simulink model "Planar_PIDC"  (R2022b)
settings: Solver=VariableStepAuto  StartTime=0.0  StopTime=40  RelTol=1e-3
values from neighbouring files (symbols this model uses):
  I = [1; 1; 1; 0.5; 0.5]*0.2    [RobDyn4link.m]
  l = [1; 1; 1; 1; 2]*0.2    [RobDyn4link.m]
  lc = l./2    [RobDyn4link.m]
  m = [1; 1; 1; 0.3; 0.3]*1    [RobDyn4link.m]
  q0 = [pi/2; -pi/4; -1*pi/6;-pi/12;0;]    [RobDyn4link.m]
  theta_max = [0.915*pi; 0.915*pi; 0.915*pi; 0.915*pi; 0.915*pi;]    [RobDyn4link.m]
  theta_min = [-0.915*pi; -0.915*pi; -0.915*pi; -0.915*pi; -0.915*pi;]    [RobDyn4link.m]
undefined symbols (not defined in the file or in its folder): DiscIntNeverNeededParam
(part 3 of 3)

== matlab function Planar_PIDC/Subsystem6/Subsystem/MATLAB Function ==
  data: theta input; M output; l input; lc input; I input; m input; Minv output
function [M,Minv] = fcn(theta,l,lc,I,m)
theta1 = theta(1); theta2 = theta(2); theta3 = theta(3); theta4 = theta(4); theta5 = theta(5);
% dtheta1 = dtheta(1); dtheta2 = dtheta(2); dtheta3 = dtheta(3); dtheta4 = dtheta(4); dtheta5 = dtheta(5);
I1 = I(1); I2 = I(2); I3 = I(3); I4 = I(4); I5 = I(5);
m1 = m(1); m2 = m(2); m3 = m(3); m4 = m(4); m5 = m(5);
l1 = l(1); l2 = l(2); l3 = l(3); l4 = l(4); l5 = l(5);
lc1 = lc(1); lc2 = lc(2); lc3 = lc(3); lc4 = lc(4); lc5 = lc(5);
% M = zeros(5,5);
% M(1,1) = I1 + I2 + I3 + I4 + I5 + l1^2*m2 + l1^2*m3 + l1^2*m4 + l2^2*m3 + l1^2*m5 + l2^2*m4 + l2^2*m5 + l3^2*m4 + l3^2*m5 + l4^2*m5 + lc1^2*m1 + lc2^2*m2 + lc3^2*m3 + lc4^2*m4 + lc5^2*m5 + 2*l1*lc5*m5*cos(theta2 + theta3 + theta4 + theta5) + 2*l1*l3*m4*cos(theta2 + theta3) + 2*l1*l3*m5*cos(theta2 + theta3) + 2*l2*l4*m5*cos(theta3 + theta4) + 2*l1*lc3*m3*cos(theta2 + theta3) + 2*l2*lc4*m4*cos(theta3 + theta4) + 2*l3*lc5*m5*cos(theta4 + theta5) + 2*l1*l2*m3*cos(theta2) + 2*l1*l2*m4*cos(theta2) + 2*l1*l2*m5*cos(theta2) + 2*l2*l3*m4*cos(theta3) + 2*l2*l3*m5*cos(theta3) + 2*l3*l4*m5*cos(theta4) + 2*l1*lc2*m2*cos(theta2) + 2*l2*lc3*m3*cos(theta3) + 2*l3*lc4*m4*cos(theta4) + 2*l4*lc5*m5*cos(theta5) + 2*l1*l4*m5*cos(theta2 + theta3 + theta4) + 2*l1*lc4*m4*cos(theta2 + theta3 + theta4) + 2*l2*lc5*m5*cos(theta3 + theta4 + theta5);
% M(1,2) = I2 + I3 + I4 + I5 + l2^2*m3 + l2^2*m4 + l2^2*m5 + l3^2*m4 + l3^2*m5 + l4^2*m5 + lc2^2*m2 + lc3^2*m3 + lc4^2*m4 + lc5^2*m5 + l1*lc5*m5*cos(theta2 + theta3 + theta4 + theta5) + l1*l3*m4*cos(theta2 + theta3) + l1*l3*m5*cos(theta2 + theta3) + 2*l2*l4*m5*cos(theta3 + theta4) + l1*lc3*m3*cos(theta2 + theta3) + 2*l2*lc4*m4*cos(theta3 + theta4) + 2*l3*lc5*m5*cos(theta4 + theta5) + l1*l2*m3*cos(theta2) + l1*l2*m4*cos(theta2) + l1*l2*m5*cos(theta2) + 2*l2*l3*m4*cos(theta3) + 2*l2*l3*m5*cos(theta3) + 2*l3*l4*m5*cos(theta4) + l1*lc2*m2*cos(theta2) + 2*l2*lc3*m3*cos(theta3) + 2*l3*lc4*m4*cos(theta4) + 2*l4*lc5*m5*cos(theta5) + l1*l4*m5*cos(theta2 + theta3 + theta4) + l1*lc4*m4*cos(theta2 + theta3 + theta4) + 2*l2*lc5*m5*cos(theta3 + theta4 + theta5);
% M(1,3) = I3 + I4 + I5 + l3^2*m4 + l3^2*m5 + l4^2*m5 + lc3^2*m3 + lc4^2*m4 + lc5^2*m5 + l1*lc5*m5*cos(theta2 + theta3 + theta4 + theta5) + l1*l3*m4*cos(theta2 + theta3) + l1*l3*m5*cos(theta2 + theta3) + l2*l4*m5*cos(theta3 + theta4) + l1*lc3*m3*cos(theta2 + theta3) + l2*lc4*m4*cos(theta3 + theta4) + 2*l3*lc5*m5*cos(theta4 + theta5) + l2*l3*m4*cos(theta3) + l2*l3*m5*cos(theta3) + 2*l3*l4*m5*cos(theta4) + l2*lc3*m3*cos(theta3) + 2*l3*lc4*m4*cos(theta4) + 2*l4*lc5*m5*cos(theta5) + l1*l4*m5*cos(theta2 + theta3 + theta4) + l1*lc4*m4*cos(theta2 + theta3 + theta4) + l2*lc5*m5*cos(theta3 + theta4 + theta5);
% M(1,4) = I4 + I5 + l4^2*m5 + lc4^2*m4 + lc5^2*m5 + l1*lc5*m5*cos(theta2 + theta3 + theta4 + theta5) + l2*l4*m5*cos(theta3 + theta4) + l2*lc4*m4*cos(theta3 + theta4) + l3*lc5*m5*cos(theta4 + theta5) + l3*l4*m5*cos(theta4) + l3*lc4*m4*cos(theta4) + 2*l4*lc5*m5*cos(theta5) + l1*l4*m5*cos(theta2 + theta3 + theta4) + l1*lc4*m4*cos(theta2 + theta3 + theta4) + l2*lc5*m5*cos(theta3 + theta4 + theta5);
% M(1,5) = I5 + lc5^2*m5 + l1*lc5*m5*cos(theta2 + theta3 + theta4 + theta5) + l3*lc5*m5*cos(theta4 + theta5) + l4*lc5*m5*cos(theta5) + l2*lc5*m5*cos(theta3 + theta4 + theta5);
% M(2,1) = M(1,1);
% M(2,2) = I2 + I3 + I4 + I5 + l2^2*m3 + l2^2*m4 + l2^2*m5 + l3^2*m4 + l3^2*m5 + l4^2*m5 + lc2^2*m2 + lc3^2*m3 + lc4^2*m4 + lc5^2*m5 + 2*l2*l4*m5*cos(theta3 + theta4) + 2*l2*lc4*m4*cos(theta3 + theta4) + 2*l3*lc5*m5*cos(theta4 + theta5) + 2*l2*l3*m4*cos(theta3) + 2*l2*l3*m5*cos(theta3) + 2*l3*l4*m5*cos(theta4) + 2*l2*lc3*m3*cos(theta3) + 2*l3*lc4*m4*cos(theta4) + 2*l4*lc5*m5*cos(theta5) + 2*l2*lc5*m5*cos(theta3 + theta4 + theta5);
% M(2,3) = I3 + I4 + I5 + l3^2*m4 + l3^2*m5 + l4^2*m5 + lc3^2*m3 + lc4^2*m4 + lc5^2*m5 + l2*l4*m5*cos(theta3 + theta4) + l2*lc4*m4*cos(theta3 + theta4) + 2*l3*lc5*m5*cos(theta4 + theta5) + l2*l3*m4*cos(theta3) + l2*l3*m5*cos(theta3) + 2*l3*l4*m5*cos(theta4) + l2*lc3*m3*cos(theta3) + 2*l3*lc4*m4*cos(theta4) + 2*l4*lc5*m5*cos(theta5) + l2*lc5*m5*cos(theta3 + theta4 + theta5);
% M(2,4) = I4 + I5 + l4^2*m5 + lc4^2*m4 + lc5^2*m5 + l2*l4*m5*cos(theta3 + theta4) + l2*lc4*m4*cos(theta3 + theta4) + l3*lc5*m5*cos(theta4 + theta5) + l3*l4*m5*cos(theta4) + l3*lc4*m4*cos(theta4) + 2*l4*lc5*m5*cos(theta5) + l2*lc5*m5*cos(theta3 + theta4 + theta5);
% M(2,5) = I5 + lc5^2*m5 + l3*lc5*m5*cos(theta4 + theta5) + l4*lc5*m5*cos(theta5) + l2*lc5*m5*cos(theta3 + theta4 + theta5);
% M(3,1) = M(1,3);
% M(3,2) = M(2,3);
% M(3,3) = I3 + I4 + I5 + l3^2*m4 + l3^2*m5 + lc3^2*m3 + lc4^2*m4 + lc4^2*m5 + lc5^2*m5 + 2*l3*lc5*m5*cos(theta4 + theta5) + 2*l3*lc4*m4*cos(theta4) + 2*l3*lc4*m5*cos(theta4) + 2*lc4*lc5*m5*cos(theta5);
% M(3,4) = m5*l4^2 + 2*m5*cos(theta5)*l4*lc5 + l3*m5*cos(theta4)*l4 + m4*lc4^2 + l3*m4*cos(theta4)*lc4 + m5*lc5^2 + l3*m5*cos(theta4 + theta5)*lc5 + I4 + I5;
% M(3,5) = I5 + lc5^2*m5 + l3*lc5*m5*cos(theta4 + theta5) + l4*lc5*m5*cos(theta5);
% M(4,1) = M(1,4);
% M(4,2) = M(2,4);
% M(4,3) = M(3,4);
% M(4,4) = m5*l4^2 + 2*m5*cos(theta5)*l4*lc5 + m4*lc4^2 + m5*lc5^2 + I4 + I5;
% M(4,5) = m5*lc5^2 + l4*m5*cos(theta5)*lc5 + I5;
% M(5,1) = M(1,5);
% M(5,2) = M(2,5);
% M(5,3) = M(3,5);
% M(5,4) = M(4,5);
% M(5,5) = m5*lc5^2 + I5;

M = [I1 + I2 + I3 + I4 + I5 + l1^2*m2 + l1^2*m3 + l1^2*m4 + l2^2*m3 + l1^2*m5 + l2^2*m4 + l2^2*m5 + l3^2*m4 + l3^2*m5 + l4^2*m5 + lc1^2*m1 + lc2^2*m2 + lc3^2*m3 + lc4^2*m4 + lc5^2*m5 + 2*l1*lc5*m5*cos(theta2 + theta3 + theta4 + theta5) + 2*l1*l3*m4*cos(theta2 + theta3) + 2*l1*l3*m5*cos(theta2 + theta3) + 2*l2*l4*m5*cos(theta3 + theta4) + 2*l1*lc3*m3*cos(theta2 + theta3) + 2*l2*lc4*m4*cos(theta3 + theta4) + 2*l3*lc5*m5*cos(theta4 + theta5) + 2*l1*l2*m3*cos(theta2) + 2*l1*l2*m4*cos(theta2) + 2*l1*l2*m5*cos(theta2) + 2*l2*l3*m4*cos(theta3) + 2*l2*l3*m5*cos(theta3) + 2*l3*l4*m5*cos(theta4) + 2*l1*lc2*m2*cos(theta2) + 2*l2*lc3*m3*cos(theta3) + 2*l3*lc4*m4*cos(theta4) + 2*l4*lc5*m5*cos(theta5) + 2*l1*l4*m5*cos(theta2 + theta3 + theta4) + 2*l1*lc4*m4*cos(theta2 + theta3 + theta4) + 2*l2*lc5*m5*cos(theta3 + theta4 + theta5), I2 + I3 + I4 + I5 + l2^2*m3 + l2^2*m4 + l2^2*m5 + l3^2*m4 + l3^2*m5 + l4^2*m5 + lc2^2*m2 + lc3^2*m3 + lc4^2*m4 + lc5^2*m5 + l1*lc5*m5*cos(theta2 + theta3 + theta4 + theta5) + l1*l3*m4*cos(theta2 + theta3) + l1*l3*m5*cos(theta2 + theta3) + 2*l2*l4*m5*cos(theta3 + theta4) + l1*lc3*m3*cos(theta2 + theta3) + 2*l2*lc4*m4*cos(theta3 + theta4) + 2*l3*lc5*m5*cos(theta4 + theta5) + l1*l2*m3*cos(theta2) + l1*l2*m4*cos(theta2) + l1*l2*m5*cos(theta2) + 2*l2*l3*m4*cos(theta3) + 2*l2*l3*m5*cos(theta3) + 2*l3*l4*m5*cos(theta4) + l1*lc2*m2*cos(theta2) + 2*l2*lc3*m3*cos(theta3) + 2*l3*lc4*m4*cos(theta4) + 2*l4*lc5*m5*cos(theta5) + l1*l4*m5*cos(theta2 + theta3 + theta4) + l1*lc4*m4*cos(theta2 + theta3 + theta4) + 2*l2*lc5*m5*cos(theta3 + theta4 + theta5), I3 + I4 + I5 + l3^2*m4 + l3^2*m5 + l4^2*m5 + lc3^2*m3 + lc4^2*m4 + lc5^2*m5 + l1*lc5*m5*cos(theta2 + theta3 + theta4 + theta5) + l1*l3*m4*cos(theta2 + theta3) + l1*l3*m5*cos(theta2 + theta3) + l2*l4*m5*cos(theta3 + theta4) + l1*lc3*m3*cos(theta2 + theta3) + l2*lc4*m4*cos(theta3 + theta4) + 2*l3*lc5*m5*cos(theta4 + theta5) + l2*l3*m4*cos(theta3) + l2*l3*m5*cos(theta3) + 2*l3*l4*m5*cos(theta4) + l2*lc3*m3*cos(theta3) + 2*l3*lc4*m4*cos(theta4) + 2*l4*lc5*m5*cos(theta5) + l1*l4*m5*cos(theta2 + theta3 + theta4) + l1*lc4*m4*cos(theta2 + theta3 + theta4) + l2*lc5*m5*cos(theta3 + theta4 + theta5), I4 + I5 + l4^2*m5 + lc4^2*m4 + lc5^2*m5 + l1*lc5*m5*cos(theta2 + theta3 + theta4 + theta5) + l2*l4*m5*cos(theta3 + theta4) + l2*lc4*m4*cos(theta3 + theta4) + l3*lc5*m5*cos(theta4 + theta5) + l3*l4*m5*cos(theta4) + l3*lc4*m4*cos(theta4) + 2*l4*lc5*m5*cos(theta5) + l1*l4*m5*cos(theta2 + theta3 + theta4) + l1*lc4*m4*cos(theta2 + theta3 + theta4) + l2*lc5*m5*cos(theta3 + theta4 + theta5), I5 + lc5^2*m5 + l1*lc5*m5*cos(theta2 + theta3 + theta4 + theta5) + l3*lc5*m5*cos(theta4 + theta5) + l4*lc5*m5*cos(theta5) + l2*lc5*m5*cos(theta3 + theta4 + theta5);
                                                                            I2 + I3 + I4 + I5 + l2^2*m3 + l2^2*m4 + l2^2*m5 + l3^2*m4 + l3^2*m5 + l4^2*m5 + lc2^2*m2 + lc3^2*m3 + lc4^2*m4 + lc5^2*m5 + l1*lc5*m5*cos(theta2 + theta3 + theta4 + theta5) + l1*l3*m4*cos(theta2 + theta3) + l1*l3*m5*cos(theta2 + theta3) + 2*l2*l4*m5*cos(theta3 + theta4) + l1*lc3*m3*cos(theta2 + theta3) + 2*l2*lc4*m4*cos(theta3 + theta4) + 2*l3*lc5*m5*cos(theta4 + theta5) + l1*l2*m3*cos(theta2) + l1*l2*m4*cos(theta2) + l1*l2*m5*cos(theta2) + 2*l2*l3*m4*cos(theta3) + 2*l2*l3*m5*cos(theta3) + 2*l3*l4*m5*cos(theta4) + l1*lc2*m2*cos(theta2) + 2*l2*lc3*m3*cos(theta3) + 2*l3*lc4*m4*cos(theta4) + 2*l4*lc5*m5*cos(theta5) + l1*l4*m5*cos(theta2 + theta3 + theta4) + l1*lc4*m4*cos(theta2 + theta3 + theta4) + 2*l2*lc5*m5*cos(theta3 + theta4 + theta5),                                                                                                                                                                                                                                                                                                                                     I2 + I3 + I4 + I5 + l2^2*m3 + l2^2*m4 + l2^2*m5 + l3^2*m4 + l3^2*m5 + l4^2*m5 + lc2^2*m2 + lc3^2*m3 + lc4^2*m4 + lc5^2*m5 + 2*l2*l4*m5*cos(theta3 + theta4) + 2*l2*lc4*m4*cos(theta3 + theta4) + 2*l3*lc5*m5*cos(theta4 + theta5) + 2*l2*l3*m4*cos(theta3) + 2*l2*l3*m5*cos(theta3) + 2*l3*l4*m5*cos(theta4) + 2*l2*lc3*m3*cos(theta3) + 2*l3*lc4*m4*cos(theta4) + 2*l4*lc5*m5*cos(theta5) + 2*l2*lc5*m5*cos(theta3 + theta4 + theta5),                                                                                                                                                                                                                                        I3 + I4 + I5 + l3^2*m4 + l3^2*m5 + l4^2*m5 + lc3^2*m3 + lc4^2*m4 + lc5^2*m5 + l2*l4*m5*cos(theta3 + theta4) + l2*lc4*m4*cos(theta3 + theta4) + 2*l3*lc5*m5*cos(theta4 + theta5) + l2*l3*m4*cos(theta3) + l2*l3*m5*cos(theta3) + 2*l3*l4*m5*cos(theta4) + l2*lc3*m3*cos(theta3) + 2*l3*lc4*m4*cos(theta4) + 2*l4*lc5*m5*cos(theta5) + l2*lc5*m5*cos(theta3 + theta4 + theta5),                                                                                                                                       I4 + I5 + l4^2*m5 + lc4^2*m4 + lc5^2*m5 + l2*l4*m5*cos(theta3 + theta4) + l2*lc4*m4*cos(theta3 + theta4) + l3*lc5*m5*cos(theta4 + theta5) + l3*l4*m5*cos(theta4) + l3*lc4*m4*cos(theta4) + 2*l4*lc5*m5*cos(theta5) + l2*lc5*m5*cos(theta3 + theta4 + theta5),                                                    I5 + lc5^2*m5 + l3*lc5*m5*cos(theta4 + theta5) + l4*lc5*m5*cos(theta5) + l2*lc5*m5*cos(theta3 + theta4 + theta5);
                                                                                                                                                                                                                                   I3 + I4 + I5 + l3^2*m4 + l3^2*m5 + l4^2*m5 + lc3^2*m3 + lc4^2*m4 + lc5^2*m5 + l1*lc5*m5*cos(theta2 + theta3 + theta4 + theta5) + l1*l3*m4*cos(theta2 + theta3) + l1*l3*m5*cos(theta2 + theta3) + l2*l4*m5*cos(theta3 + theta4) + l1*lc3*m3*cos(theta2 + theta3) + l2*lc4*m4*cos(theta3 + theta4) + 2*l3*lc5*m5*cos(theta4 + theta5) + l2*l3*m4*cos(theta3) + l2*l3*m5*cos(theta3) + 2*l3*l4*m5*cos(theta4) + l2*lc3*m3*cos(theta3) + 2*l3*lc4*m4*cos(theta4) + 2*l4*lc5*m5*cos(theta5) + l1*l4*m5*cos(theta2 + theta3 + theta4) + l1*lc4*m4*cos(theta2 + theta3 + theta4) + l2*lc5*m5*cos(theta3 + theta4 + theta5),                                                                                                                                                                                                                                                                                                                                                                                               I3 + I4 + I5 + l3^2*m4 + l3^2*m5 + l4^2*m5 + lc3^2*m3 + lc4^2*m4 + lc5^2*m5 + l2*l4*m5*cos(theta3 + theta4) + l2*lc4*m4*cos(theta3 + theta4) + 2*l3*lc5*m5*cos(theta4 + theta5) + l2*l3*m4*cos(theta3) + l2*l3*m5*cos(theta3) + 2*l3*l4*m5*cos(theta4) + l2*lc3*m3*cos(theta3) + 2*l3*lc4*m4*cos(theta4) + 2*l4*lc5*m5*cos(theta5) + l2*lc5*m5*cos(theta3 + theta4 + theta5),                                                                                                                                                                                                                                                                                                                                                                                                                         I3 + I4 + I5 + l3^2*m4 + l3^2*m5 + l4^2*m5 + lc3^2*m3 + lc4^2*m4 + lc5^2*m5 + 2*l3*lc5*m5*cos(theta4 + theta5) + 2*l3*l4*m5*cos(theta4) + 2*l3*lc4*m4*cos(theta4) + 2*l4*lc5*m5*cos(theta5),                                                                                                                                                                                                                                                  m5*l4^2 + 2*m5*cos(theta5)*l4*lc5 + l3*m5*cos(theta4)*l4 + m4*lc4^2 + l3*m4*cos(theta4)*lc4 + m5*lc5^2 + l3*m5*cos(theta4 + theta5)*lc5 + I4 + I5,                                                                                              I5 + lc5^2*m5 + l3*lc5*m5*cos(theta4 + theta5) + l4*lc5*m5*cos(theta5);
                                                                                                                                                                                                                                                                                                                                                                                                                                                    I4 + I5 + l4^2*m5 + lc4^2*m4 + lc5^2*m5 + l1*lc5*m5*cos(theta2 + theta3 + theta4 + theta5) + l2*l4*m5*cos(theta3 + theta4) + l2*lc4*m4*cos(theta3 + theta4) + l3*lc5*m5*cos(theta4 + theta5) + l3*l4*m5*cos(theta4) + l3*lc4*m4*cos(theta4) + 2*l4*lc5*m5*cos(theta5) + l1*l4*m5*cos(theta2 + theta3 + theta4) + l1*lc4*m4*cos(theta2 + theta3 + theta4) + l2*lc5*m5*cos(theta3 + theta4 + theta5),                                                                                                                                                                                                                                                                                                                                                                                                                                                                                                               I4 + I5 + l4^2*m5 + lc4^2*m4 + lc5^2*m5 + l2*l4*m5*cos(theta3 + theta4) + l2*lc4*m4*cos(theta3 + theta4) + l3*lc5*m5*cos(theta4 + theta5) + l3*l4*m5*cos(theta4) + l3*lc4*m4*cos(theta4) + 2*l4*lc5*m5*cos(theta5) + l2*lc5*m5*cos(theta3 + theta4 + theta5),                                                                                                                                                                                                                                                                                                                                                                                                                                                                   m5*l4^2 + 2*m5*cos(theta5)*l4*lc5 + l3*m5*cos(theta4)*l4 + m4*lc4^2 + l3*m4*cos(theta4)*lc4 + m5*lc5^2 + l3*m5*cos(theta4 + theta5)*lc5 + I4 + I5,                                                                                                                                                                                                                                                                                                                                  m5*l4^2 + 2*m5*cos(theta5)*l4*lc5 + m4*lc4^2 + m5*lc5^2 + I4 + I5,                                                                                                                               m5*lc5^2 + l4*m5*cos(theta5)*lc5 + I5;
                                                                                                                                                                                                                                                                                                                                                                                                                                                                                                                                                                                                                                                                                   I5 + lc5^2*m5 + l1*lc5*m5*cos(theta2 + theta3 + theta4 + theta5) + l3*lc5*m5*cos(theta4 + theta5) + l4*lc5*m5*cos(theta5) + l2*lc5*m5*cos(theta3 + theta4 + theta5),                                                                                                                                                                                                                                                                                                                                                                                                                                                                                                                                                                                                                                                           I5 + lc5^2*m5 + l3*lc5*m5*cos(theta4 + theta5) + l4*lc5*m5*cos(theta5) + l2*lc5*m5*cos(theta3 + theta4 + theta5),                                                                                                                                                                                                                                                                                                                                                                                                                                                                                                                                              I5 + lc5^2*m5 + l3*lc5*m5*cos(theta4 + theta5) + l4*lc5*m5*cos(theta5),                                                                                                                                                                                                                                                                                                                                                              m5*lc5^2 + l4*m5*cos(theta5)*lc5 + I5,                                                                                                                                                       m5*lc5^2 + I5;];

Minv = inv(M);

== matlab function Planar_PIDC/Subsystem6/Subsystem2/MATLAB Function ==
  data: theta input; G output; m input; l input; lc input
function G = fcn(theta,m,l,lc)
theta1 = theta(1); theta2 = theta(2); theta3 = theta(3); theta4 = theta(4); theta5 = theta(5);
% dtheta1 = dtheta(1); dtheta2 = dtheta(2); dtheta3 = dtheta(3); dtheta4 = dtheta(4); dtheta5 = dtheta(5);
% I1 = I(1); I2 = I(2); I3 = I(3); I4 = I(4); I5 = I(5);
m1 = m(1); m2 = m(2); m3 = m(3); m4 = m(4); m5 = m(5);
l1 = l(1); l2 = l(2); l3 = l(3); l4 = l(4); l5 = l(5);
lc1 = lc(1); lc2 = lc(2); lc3 = lc(3); lc4 = lc(4); lc5 = lc(5);
g = 9.81;

G = [g*l4*m4*cos(theta1 + theta2 + theta3 + theta4) + g*lc4*m4*cos(theta1 + theta2 + theta3 + theta4) + g*l2*m3*cos(theta1 + theta2) + 2*g*l2*m4*cos(theta1 + theta2) + g*lc2*m2*cos(theta1 + theta2) + g*l1*m2*cos(theta1) + g*l1*m3*cos(theta1) + 2*g*l1*m4*cos(theta1) + g*lc1*m1*cos(theta1) + g*lc5*m4*cos(theta1 + theta2 + theta3 + theta4 + theta5) + 2*g*l3*m4*cos(theta1 + theta2 + theta3) + g*lc3*m3*cos(theta1 + theta2 + theta3);
                                                                                           g*l4*m4*cos(theta1 + theta2 + theta3 + theta4) + g*lc4*m4*cos(theta1 + theta2 + theta3 + theta4) + g*l2*m3*cos(theta1 + theta2) + 2*g*l2*m4*cos(theta1 + theta2) + g*lc2*m2*cos(theta1 + theta2) + g*lc5*m4*cos(theta1 + theta2 + theta3 + theta4 + theta5) + 2*g*l3*m4*cos(theta1 + theta2 + theta3) + g*lc3*m3*cos(theta1 + theta2 + theta3);
                                                                                                                                                                                           g*l4*m4*cos(theta1 + theta2 + theta3 + theta4) + g*lc4*m4*cos(theta1 + theta2 + theta3 + theta4) + g*lc5*m4*cos(theta1 + theta2 + theta3 + theta4 + theta5) + 2*g*l3*m4*cos(theta1 + theta2 + theta3) + g*lc3*m3*cos(theta1 + theta2 + theta3);
                                                                                                                                                                                                                                                                                 g*m4*(l4*cos(theta1 + theta2 + theta3 + theta4) + lc5*cos(theta1 + theta2 + theta3 + theta4 + theta5)) + g*lc4*m4*cos(theta1 + theta2 + theta3 + theta4);
                                                                                                                                                                                                                                                                                                                                                                                 g*lc5*m4*cos(theta1 + theta2 + theta3 + theta4 + theta5)];

== matlab function Planar_PIDC/Subsystem6/Subsystem4/MATLAB Function ==
  data: theta input; J5e output; l input; J5 output; J4e output; J4 output
function [J5e,J5,J4e,J4] = fcn(theta,l)
l1 = l(1); l2 = l(2); l3 = l(3); l4 = l(4); l5 = l(5);
theta1 = theta(1); theta2 = theta(2); theta3 = theta(3); theta4 = theta(4); theta5 = theta(5);



J5e = [- l4*sin(theta1 + theta2 + theta3 + theta4) - l2*sin(theta1 + theta2) - l1*sin(theta1) - l5*sin(theta1 + theta2 + theta3 + theta4 + theta5) - l3*sin(theta1 + theta2 + theta3), - l4*sin(theta1 + theta2 + theta3 + theta4) - l2*sin(theta1 + theta2) - l5*sin(theta1 + theta2 + theta3 + theta4 + theta5) - l3*sin(theta1 + theta2 + theta3), - l4*sin(theta1 + theta2 + theta3 + theta4) - l5*sin(theta1 + theta2 + theta3 + theta4 + theta5) - l3*sin(theta1 + theta2 + theta3), - l4*sin(theta1 + theta2 + theta3 + theta4) - l5*sin(theta1 + theta2 + theta3 + theta4 + theta5), -l5*sin(theta1 + theta2 + theta3 + theta4 + theta5);
  l4*cos(theta1 + theta2 + theta3 + theta4) + l2*cos(theta1 + theta2) + l1*cos(theta1) + l5*cos(theta1 + theta2 + theta3 + theta4 + theta5) + l3*cos(theta1 + theta2 + theta3),   l4*cos(theta1 + theta2 + theta3 + theta4) + l2*cos(theta1 + theta2) + l5*cos(theta1 + theta2 + theta3 + theta4 + theta5) + l3*cos(theta1 + theta2 + theta3),   l4*cos(theta1 + theta2 + theta3 + theta4) + l5*cos(theta1 + theta2 + theta3 + theta4 + theta5) + l3*cos(theta1 + theta2 + theta3),   l4*cos(theta1 + theta2 + theta3 + theta4) + l5*cos(theta1 + theta2 + theta3 + theta4 + theta5),  l5*cos(theta1 + theta2 + theta3 + theta4 + theta5);
                                                                                                                                                                             1,                                                                                                                                                             1,                                                                                                                                   1,                                                                                                1,                                                   1;];
J5 =  [- l4*sin(theta1 + theta2 + theta3 + theta4) - l2*sin(theta1 + theta2) - l1*sin(theta1) - l3*sin(theta1 + theta2 + theta3), - l4*sin(theta1 + theta2 + theta3 + theta4) - l2*sin(theta1 + theta2) - l3*sin(theta1 + theta2 + theta3), - l4*sin(theta1 + theta2 + theta3 + theta4) - l3*sin(theta1 + theta2 + theta3), -l4*sin(theta1 + theta2 + theta3 + theta4), 0;
  l4*cos(theta1 + theta2 + theta3 + theta4) + l2*cos(theta1 + theta2) + l1*cos(theta1) + l3*cos(theta1 + theta2 + theta3),   l4*cos(theta1 + theta2 + theta3 + theta4) + l2*cos(theta1 + theta2) + l3*cos(theta1 + theta2 + theta3),   l4*cos(theta1 + theta2 + theta3 + theta4) + l3*cos(theta1 + theta2 + theta3),  l4*cos(theta1 + theta2 + theta3 + theta4), 0;
                                                                                                                        1,                                                                                                        1,                                                                              1,                                          1, 1];
J4e = [- l4*sin(theta1 + theta2 + theta3 + theta4) - l2*sin(theta1 + theta2) - l1*sin(theta1) - l3*sin(theta1 + theta2 + theta3), - l4*sin(theta1 + theta2 + theta3 + theta4) - l2*sin(theta1 + theta2) - l3*sin(theta1 + theta2 + theta3), - l4*sin(theta1 + theta2 + theta3 + theta4) - l3*sin(theta1 + theta2 + theta3), -l4*sin(theta1 + theta2 + theta3 + theta4), 0;
  l4*cos(theta1 + theta2 + theta3 + theta4) + l2*cos(theta1 + theta2) + l1*cos(theta1) + l3*cos(theta1 + theta2 + theta3),   l4*cos(theta1 + theta2 + theta3 + theta4) + l2*cos(theta1 + theta2) + l3*cos(theta1 + theta2 + theta3),   l4*cos(theta1 + theta2 + theta3 + theta4) + l3*cos(theta1 + theta2 + theta3),  l4*cos(theta1 + theta2 + theta3 + theta4), 0;
                                                                                                                        1,                                                                                                        1,                                                                              1,                                          1, 0];
J4 = [- l2*sin(theta1 + theta2) - l1*sin(theta1) - l3*sin(theta1 + theta2 + theta3), - l2*sin(theta1 + theta2) - l3*sin(theta1 + theta2 + theta3), -l3*sin(theta1 + theta2 + theta3), 0, 0;
  l2*cos(theta1 + theta2) + l1*cos(theta1) + l3*cos(theta1 + theta2 + theta3),   l2*cos(theta1 + theta2) + l3*cos(theta1 + theta2 + theta3),  l3*cos(theta1 + theta2 + theta3), 0, 0;
                                                                            1,                                                            1,                                 1, 1, 0];

== matlab function Planar_PIDC/Subsystem6/Subsystem5/MATLAB Function ==
  data: xc input; xee input; xee_0 output; yee input; yee_0 output
function [xee_0,yee_0] = fcn(xc, xee, yee)

xee_0 = [0;xee;xc(1)];
yee_0 = [0;yee;xc(2)];

== matlab function Planar_PIDC/Subsystem6/Subsystem5/MATLAB Function1 ==
  data: xe output; theta input; ye output; l input; Xee output; X5 output
function [xe,ye,Xee,X5] = fcn(theta,l)
theta1 = theta(1); theta2 = theta(2); theta3 = theta(3); theta4 = theta(4); theta5 = theta(5);
% dtheta1 = dtheta(1); dtheta2 = dtheta(2); dtheta3 = dtheta(3); dtheta4 = dtheta(4); dtheta5 = dtheta(5);
% I1 = I(1); I2 = I(2); I3 = I(3); I4 = I(4); I5 = I(5);
% m1 = m(1); m2 = m(2); m3 = m(3); m4 = m(4); m5 = m(5);
l1 = l(1); l2 = l(2); l3 = l(3); l4 = l(4); l5 = l(5);
% lc1 = lc(1); lc2 = lc(2); lc3 = lc(3); lc4 = lc(4); lc5 = lc(5);

x1e = l1 * cos(theta1);
y1e = l1 * sin(theta1);

x2e = l1 * cos(theta1) + l2 * cos(theta1 + theta2);
y2e = l1 * sin(theta1) + l2 * sin(theta1 + theta2);

x3e = l1 * cos(theta1) + l2 * cos(theta1 + theta2) + l3 * cos(theta1 + theta2 + theta3);
y3e = l1 * sin(theta1) + l2 * sin(theta1 + theta2) + l3 * sin(theta1 + theta2 + theta3);

x4e = l1 * cos(theta1) + l2 * cos(theta1 + theta2) + l3 * cos(theta1 + theta2 + theta3) + l4 * cos(theta1 + theta2 + theta3 + theta4);
y4e = l1 * sin(theta1) + l2 * sin(theta1 + theta2) + l3 * sin(theta1 + theta2 + theta3) + l4 * sin(theta1 + theta2 + theta3 + theta4);

x5e = l1 * cos(theta1) + l2 * cos(theta1 + theta2) + l3 * cos(theta1 + theta2 + theta3) + l4 * cos(theta1 + theta2 + theta3 + theta4) + l5 * cos(theta1 + theta2 + theta3 + theta4 + theta5);
y5e = l1 * sin(theta1) + l2 * sin(theta1 + theta2) + l3 * sin(theta1 + theta2 + theta3) + l4 * sin(theta1 + theta2 + theta3 + theta4) + l5 * sin(theta1 + theta2 + theta3 + theta4 + theta5);

xe = [x1e;x2e;x3e;x4e;x5e];
ye = [y1e;y2e;y3e;y4e;y5e];

Xee = [x5e;y5e;theta1+theta2+theta3+theta4+theta5];

x1 = 0;
y1 = 0;

x2 = l1 * cos(theta1);
y2 = l1 * sin(theta1);

x3 = l1 * cos(theta1) + l2 * cos(theta1 + theta2);
y3 = l1 * sin(theta1) + l2 * sin(theta1 + theta2);

x4 = l1 * cos(theta1) + l2 * cos(theta1 + theta2) + l3 * cos(theta1 + theta2 + theta3);
y4 = l1 * sin(theta1) + l2 * sin(theta1 + theta2) + l3 * sin(theta1 + theta2 + theta3);

x5 = l1 * cos(theta1) + l2 * cos(theta1 + theta2) + l3 * cos(theta1 + theta2 + theta3) + l4 * cos(theta1 + theta2 + theta3 + theta4);
y5 = l1 * sin(theta1) + l2 * sin(theta1 + theta2) + l3 * sin(theta1 + theta2 + theta3) + l4 * sin(theta1 + theta2 + theta3 + theta4);

x = [x1,x2,x3,x4,x5]';
y = [y1,y2,y3,y4,y5]';
X5 = [x5;y5;theta1+theta2+theta3+theta4+theta5];

== matlab function Planar_PIDC/Subsystem3/MATLAB Function2 ==
  data: Jc input; Jc_dot input; tau output; Sf output; M input; Jee input; Jee_dot input; C input; thetadot input; xdes input; xdes_dot input; xdes_ddot input; xee input; xee_dot input; xc_proj input; Vr input; Vcf input; tau_ext input; Sc output; Stotal output; tau_ext_s input; tau_ext_dot output
function [tau,Sf,Sc,Stotal,tau_ext_dot]= fcn(Jc,Jc_dot,M,Jee,Jee_dot,C,thetadot,xdes,xdes_dot,xdes_ddot,xee,xee_dot, xc_proj, Vr, Vcf,tau_ext,tau_ext_s)
Jc_pinv = Jc'/(Jc*Jc');
Jc_sharp = inv(M)*Jc'/(Jc*inv(M)*Jc');

P = eye(5) - Jc_pinv*Jc;
% P = eye(5) - Jc'*Jc_sharp';

xee = xee(1:2);
xee_dot = Jee*thetadot;
xee_dot = xee_dot(1:2);
Jee = Jee(1:2,:);
Jee_dot = Jee_dot(1:2,:);
Jz = Jee;
Jz_dot = Jee_dot;
xz = xee;
xz_ddot = xee;


Kpe = 100;
Kp = eye(2) * Kpe; 
Kd = eye(2) * sqrt(Kpe)*2; 

%% orthogonal decomposition approach
xcmd_ddot = xdes_ddot + Kd*(xdes_dot - xee_dot) + Kp*(xdes - xee);
Jee_sharp = inv(M)*Jee'/(Jee*inv(M)*Jee');
Jee_pinv = Jee'/(Jee*Jee');
qcmd_ddot = Jee_sharp*(xcmd_ddot - Jee_dot*thetadot);
% tau = P*(M*qcmd_ddot+C*thetadot);

P_pinv = P'/(P*P'+1e-5*eye(5));
% Jc_sharp = inv(M)*Jc'/(Jc*inv(M)*Jc');

Mc = P*M + eye(5) - P;
Lambda_c = inv(Jee/Mc*P*Jee');
H_c = Lambda_c*(Jee/Mc*P*C*thetadot - (Jee_dot + Jee/Mc*(-Jc_pinv*Jc_dot))*thetadot);
F_cosf = Lambda_c*(xdes_ddot + Kd*(xdes_dot - xee_dot) + Kp*(xdes - xee)) + H_c; % good one
% F_cosf =  Kd*(- xee_dot) + Kp*(xdes - xee) + H_c; % passivity test


Kpc = 1000;
xc_des_ddot = 0 + (2*sqrt(Kpc)*(0-Vr) + Kpc*(0 - xc_proj));
tau_c = M*Jc_sharp*(xc_des_ddot - Vcf + Jc_dot*thetadot) + C*thetadot; % good one
% tau_c = Jc_sharp*(xc_des_ddot - Vcf + Jc_dot*thetadot) + C*thetadot; % test passivity

% tau_c = Jc'*(xc_des_ddot - Vcf + Jc_dot*thetadot) + C*thetadot;

Mrcm = (eye(5) - P)*M + P;
Lambda_rcm = inv(Jc/Mrcm*Jc'); H_rcm = Lambda_rcm*(Jc/M*(C )*thetadot - Jc_dot*thetadot + Vcf);
Frcm_des = 2*sqrt(Kpc)*(0-Vr) + Kpc*(0 - xc_proj) + H_rcm;
F_rcm = Frcm_des;
tau_rcm = Jc'*F_rcm;  % use it together with tau_osf, they are correspondent

Lambda = inv(Jee/M*Jee'); h = Lambda*(Jee/M*C*thetadot - Jee_dot*thetadot);
F_osf = Lambda*xcmd_ddot + h;

tau_f_osf = Jee'*F_osf;
tau_f_cosf = Jee'*F_cosf;
tau_f_pidc = P*(M*P*qcmd_ddot+C*thetadot);

%% multi-priority control


J1 = Jee;   J1_dot = Jee_dot;  x1cmd_ddot = xcmd_ddot;
J2 = Jc; J2_dot = Jc_dot; x2cmd_ddot = xc_des_ddot;

% J1 = Jc;   J1_dot = Jc_dot;  x1cmd_ddot = xc_des_ddot;
% J2 = Jee; J2_dot = Jee_dot; x2cmd_ddot = xcmd_ddot;


J1_pinv = J1'/(J1*J1');
N1 = eye(5) - J1_pinv*J1;


J2_bar = J2*N1;
J2_bar_pinv = J2_bar'/(J2_bar*J2_bar');

q1cmd_ddot = J1_pinv*(x1cmd_ddot - J1_dot*thetadot);
q2cmd_ddot = J2_bar_pinv*(x2cmd_ddot - J2_dot*thetadot - J2*q1cmd_ddot);

tau_multi = M*(q1cmd_ddot+q2cmd_ddot) + C*thetadot;

%% passivity based approach
Ps = eye(2)*25;
s = xdes_dot - xee_dot + Ps*(xdes - xee);
K = eye(2)*80;
tau_parallel = Jee'*((xdes_ddot + Ps*(xdes_dot - xee_dot) + K*s) - 1*Jee_sharp'*tau_ext_s);
tau_perp = Jc'*F_rcm;
Gamma_f = eye(5)*0.0125;
f_x = 1/(1+ norm(xdes - xee))*(xdes - xee);
tau_ext_dot = -inv(Gamma_f)*Jee_sharp*(xdes_dot - xee_dot  + 5*f_x);
tau =  (eye(5) - P)*tau_perp+ (P)*tau_parallel - 0*tau_ext_s;

%% control law composition
% tau = (eye(5) - P)*tau_c+ (P)*tau_f_cosf - 0*tau_ext;
% tau = tau_multi;


%% compute some passivity related metrics
Skf = (xee_dot - xdes_dot)'*Lambda_c*(xee_dot - xdes_dot);
Skc = Vr'*Lambda_rcm*Vr;
Vf = (xdes - xee)'*Kp*(xdes - xee);
Vc = (0 - xc_proj)'*Kpc*(0 - xc_proj);
Sf = 0.5*(Skf + Vf);
Sc = 0.5*(Skc + Vc);
% Stotal = 0.5*(Sf + Sc);
Stotal = 0.5*thetadot'*M*thetadot +  Vf + Vc;


%% embedded nullspace impedance control
% not really compatible in practice....

% Psharp = eye(5) - Jc'*Jc_sharp';
% [V1,D1] = eig(P);
% Z1 = V1(:,2:end);
% J3_prime = Jee*Z1;
% J3_pm = J3_prime(:,1:2);
% J3_pr = J3_prime(:,3:4);
% Z3 = [-J3_pr'/J3_pm', eye(2)];
% Lambda_P = inv(Jz/Mc*P*Jz');
% Lambda_3 = (J3_prime*Lambda_P)
